simulink subsystem "Rectifier"  (R2023b)
settings: Solver=VariableStepAuto  StartTime=0.0  StopTime=10.0  RelTol=1e-3
libraries: fl_lib x4
settings Model: Creator=torenarginteanu  LastModifiedBy=torenarginteanu

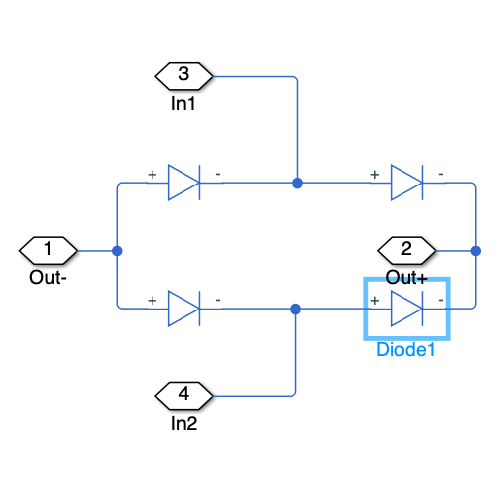
[thumbnail: Simulink's stored preview of the top-level diagram]
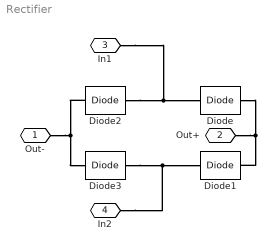
== system Rectifier ==
  Diode{,1..3} (4 alike) : fl_lib/Electrical/Electrical Elements/Diode  Vf=1.2 V  Ron=0.3 Ohm  Goff=1e-8 1/Ohm  i_specify=off  i_priority=None  i=0 A  i_nominal_specify=off  i_nominal_unit=A  i_nominal_value=1  v_specify=off  v_priority=None  v=0 V  v_nominal_specify=off  v_nominal_unit=V  v_nominal_value=1
  Out- : PMIOPort  Side=Left
  Out+ : PMIOPort  Port=2  Side=Left
  In1 : PMIOPort  Port=3  Side=Left
  In2 : PMIOPort  Port=4  Side=Left
  connections:
  Diode/RConn1 -- Out+/RConn1 -- Diode1/RConn1
  Diode2/LConn1 -- Out-/RConn1 -- Diode3/LConn1
  Diode3/RConn1 -- In2/RConn1 -- Diode1/LConn1
  Diode2/RConn1 -- In1/RConn1 -- Diode/LConn1
